simulink model "gain_scheduling"  (R2022a)
settings: Solver=VariableStepAuto  StartTime=0.0  StopTime=7  RelTol=1e-3
values from neighbouring files (symbols this model uses):
  A_g = [    -0.4340     , 0.9473 ... (first row only)    [gains_sched.m]
  B_g = [ -0.0009 ... (first row only)    [gains_sched.m]
  C_g = [57.2958, 0; 0, 57.2958]    [gains_sched.m]
  D_g = [0; 0]    [gains_sched.m]
  K_gains_sched = place(A_g, B_g, p_g)    [gains_sched.m]
settings Model: Creator=mihai  LastModifiedBy=mihai

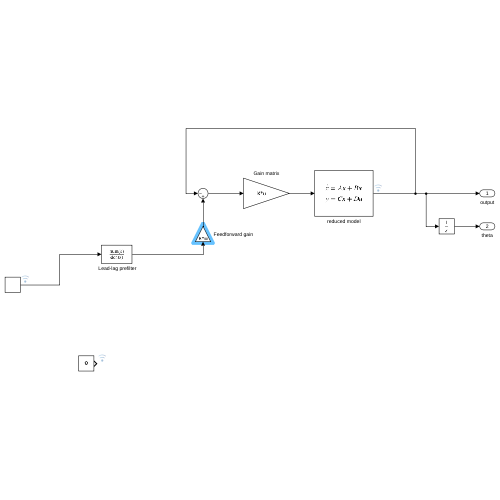
[thumbnail: Simulink's stored preview of the top-level diagram]
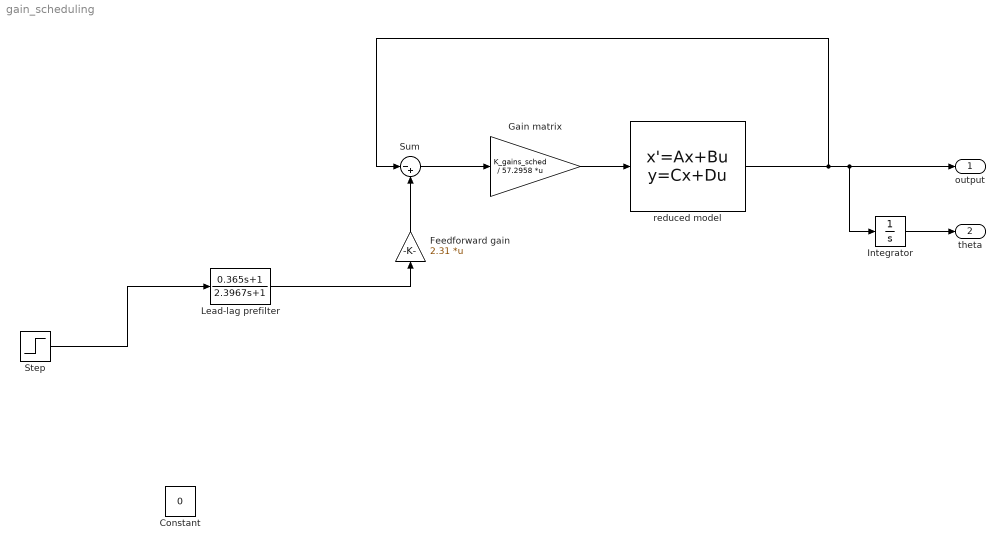
== system gain_scheduling ==
  " Lead-lag prefilter" : TransferFcn  Numerator=[0.365, 1]  Denominator=[2.3967, 1]
  Constant : Constant  Value=0
  Feedforward gain : Gain  Gain=2.31  Multiplication=Matrix(K*u)
  Gain matrix : Gain  Gain=K_gains_sched / 57.2958  Multiplication=Matrix(K*u)
  Integrator : Integrator
  Step : Step  Time=0  OutDataTypeStr=Inherit: Inherit via back propagation  SampleTime=0
  Sum : Sum  Inputs=|-+
  reduced model : StateSpace  A=A_g  B=B_g  C=C_g  D=D_g  InitialCondition=0
  output : Outport
  theta : Outport  Port=2
  wires:
  Gain matrix/1 -> reduced model/1
  Sum/1 -> Gain matrix/1
  Step/1 -> " Lead-lag prefilter"/1
  " Lead-lag prefilter"/1 -> Feedforward gain/1
  Feedforward gain/1 -> Sum/2
  Integrator/1 -> theta/1
  reduced model/1 -> Sum/1, Integrator/1, output/1
